simulink model "control_02_flightpath"  (R2020a)
settings: Solver=FixedStepAuto  StartTime=0.0  StopTime=10.0  RelTol=1e-3
model workspace (MAT data in the model file):
  chi = 0.7
  omega = 100
libraries: discretizing x5, simulink x3
settings Model: Creator=Bayram  LastModifiedBy=Julius

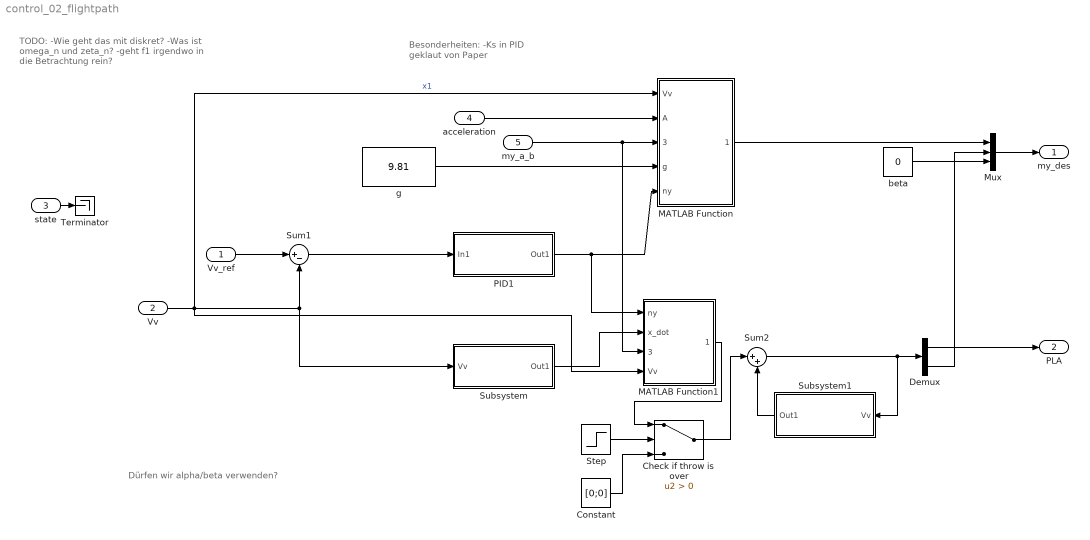
== system control_02_flightpath ==
  note: Dürfen wir alpha/beta verwenden?
  note: Besonderheiten:
      | -Ks in PID geklaut von Paper
  note: TODO:
      | -Wie geht das mit diskret?
      | -Was ist omega_n und zeta_n?
      | -geht f1 irgendwo in die Betrachtung rein?
  Vv_ref : Inport  PortDimensions=3
  Vv : Inport  Port=2  OutDataTypeStr=single  PortDimensions=3
  state : Inport  Port=3  OutDataTypeStr=Bus:fmBus
  acceleration : Inport  Port=4  OutDataTypeStr=single  PortDimensions=3
  my_a_b : Inport  Port=5  OutDataTypeStr=single  PortDimensions=3
  Check if throw is over : Switch  Criteria=u2 > Threshold
  Constant : Constant  Value=[0;0]  OutDataTypeStr=single
  Demux : Demux  Outputs=2
  MATLAB Function : MATLAB Function  TreatAsAtomicUnit=on
  MATLAB Function1 : MATLAB Function  TreatAsAtomicUnit=on
  Mux : Mux  Inputs=3
  PID1 : Subsystem
  Step : Step  Time=7  SampleTime=0
  Subsystem : Subsystem
  Subsystem1 : Subsystem
  Sum1 : Sum  Inputs=|+-
  Sum2 : Sum  Inputs=|++  AccumDataTypeStr=single  OutDataTypeStr=single
  Terminator : Terminator
  beta : Constant  Value=0  OutDataTypeStr=single
  g : Constant  Value=9.81  OutDataTypeStr=double
  my_des : Outport  OutDataTypeStr=single  PortDimensions=3
  PLA : Outport  Port=2  OutDataTypeStr=single  PortDimensions=1
  wires:
  state/1 -> Terminator/1
  MATLAB Function/1(mu_des) -> Mux/1
  Sum2/1 -> Demux/1, Subsystem1/1(Vv)
  Sum1/1 -> PID1/1(In1)
  acceleration/1 -> MATLAB Function/2(A)
  g/1 -> MATLAB Function/4(g)
  PID1/1(Out1) -> MATLAB Function1/1(ny), MATLAB Function/5(ny)
  Vv_ref/1 -> Sum1/1
  Vv/1 -> MATLAB Function/1(Vv), MATLAB Function1/4(Vv), Subsystem/1(Vv), Sum1/2  "x1"
  Subsystem/1(Out1) -> MATLAB Function1/2(x_dot)
  Subsystem1/1(Out1) -> Sum2/2
  my_a_b/1 -> MATLAB Function1/3(my_a_b), MATLAB Function/3(my_a_b)
  beta/1 -> Mux/3
  Mux/1 -> my_des/1
  Demux/1 -> PLA/1
  Demux/2 -> Mux/2
  Constant/1 -> Check if throw is over/3
  Step/1 -> Check if throw is over/2
  MATLAB Function1/1(Delta_x) -> Check if throw is over/1
  Check if throw is over/1 -> Sum2/1

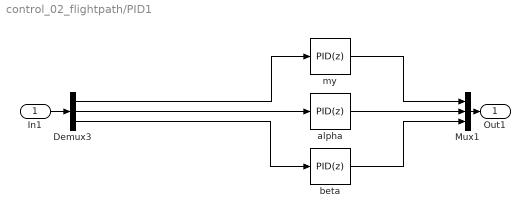
== system control_02_flightpath/PID1 ==
  In1 : Inport
  Demux3 : Demux  Outputs=3
  Mux1 : Mux  Inputs=3
  alpha : simulink/Continuous/PID Controller  Controller=PID  Form=Parallel  TimeDomain=Discrete-time  UseExternalTs=off  SampleTime=-1  IntegratorMethod=Forward Euler  FilterMethod=Forward Euler  ControllerParametersSource=internal  P=1  I=0  D=0  UseFilter=on  N=100  TunerSelectOption=Transfer Function Based (PID Tuner App)  InitialConditionSource=internal  InitialConditionForIntegrator=0  InitialConditionForFilter=0  DifferentiatorICPrevScaledInput=0  ExternalReset=none  TrackingMode=off  Kt=1  LimitOutput=off  UpperSaturationLimit=inf  LowerSaturationLimit=-inf  LinearizeAsGain=off  AntiWindupMode=none  Kb=1  POutMin=[]  POutMax=[]  IOutMin=[]  IOutMax=[]  DOutMin=[]  DOutMax=[]  NOutMin=[]  NOutMax=[]  SumOutMin=[]  SumOutMax=[]  SaturationOutMin=[]  SaturationOutMax=[]  PParamMin=[]  PParamMax=[]  IParamMin=[]  IParamMax=[]  DParamMin=[]  DParamMax=[]  NParamMin=[]  NParamMax=[]  KbParamMin=[]  KbParamMax=[]  KtParamMin=[]  KtParamMax=[]  KbOutMin=[]  KbOutMax=[]  KtOutMin=[]  KtOutMax=[]  IntegratorOutMin=[]  IntegratorOutMax=[]  FilterOutMin=[]  FilterOutMax=[]  SumI1OutMin=[]  SumI1OutMax=[]  SumI2OutMin=[]  SumI2OutMax=[]  SumI3OutMin=[]  SumI3OutMax=[]  SumI4OutMin=[]  SumI4OutMax=[]  SumDOutMin=[]  SumDOutMax=[]  DifferentiatorOutMin=[]  DifferentiatorOutMax=[]  FilterDiffOutCoefMin=[]  FilterDiffOutCoefMax=[]  ReciprocalOutMin=[]  ReciprocalOutMax=[]  SumDenOutMin=[]  SumDenOutMax=[]  SumNumOutMin=[]  SumNumOutMax=[]  DivideOutMin=[]  DivideOutMax=[]  UdiffTsProdOutMin=[]  UdiffTsProdOutMax=[]  NTsProdOutMin=[]  NTsProdOutMax=[]  UintegralTsProdOutMin=[]  UintegralTsProdOutMax=[]  UngainTsProdOutMin=[]  UngainTsProdOutMax=[]  IntegratorContinuousStateAttributes=''  IntegratorStateMustResolveToSignalObject=off  IntegratorRTWStateStorageClass=Auto  FilterContinuousStateAttributes=''  FilterStateMustResolveToSignalObject=off  FilterRTWStateStorageClass=Auto  ParallelPVariant=InternalParameters  IdealPVariant=Disabled  IVariant=InternalParameters  DVariant=InternalParameters  IntegratorVariant=Discrete  SatVariant=Disabled  AWVariant=Passthrough  PCopyVariant=Disabled  TRVariant=Disabled  FdbkBlocksVariant=Forward  IdealPFdbkVariant=Disabled  SatFdbkVariant=Disabled  DerivativeFilterVariant=ForwardEulerFilter  NVariant=InternalParameters  NCopyVariant=Disabled  FilterICVariant=InternalICsFilter  IntegratorICVariant=InternalICs  ExternalResetVariant=Disabled  TRSumVariant=Passthrough  SumFdbkVariant=Disabled  SumVariant=Sum_PID  TsampFilterVariant=InternalTs  TsampNgainVariant=Passthrough  TsampIntegralVariant=Passthrough
  beta : simulink/Continuous/PID Controller  Controller=PID  Form=Parallel  TimeDomain=Discrete-time  UseExternalTs=off  SampleTime=-1  IntegratorMethod=Forward Euler  FilterMethod=Forward Euler  ControllerParametersSource=internal  P=1  I=0  D=0  UseFilter=on  N=100  TunerSelectOption=Transfer Function Based (PID Tuner App)  InitialConditionSource=internal  InitialConditionForIntegrator=0  InitialConditionForFilter=0  DifferentiatorICPrevScaledInput=0  ExternalReset=none  TrackingMode=off  Kt=1  LimitOutput=off  UpperSaturationLimit=inf  LowerSaturationLimit=-inf  LinearizeAsGain=off  AntiWindupMode=none  Kb=1  POutMin=[]  POutMax=[]  IOutMin=[]  IOutMax=[]  DOutMin=[]  DOutMax=[]  NOutMin=[]  NOutMax=[]  SumOutMin=[]  SumOutMax=[]  SaturationOutMin=[]  SaturationOutMax=[]  PParamMin=[]  PParamMax=[]  IParamMin=[]  IParamMax=[]  DParamMin=[]  DParamMax=[]  NParamMin=[]  NParamMax=[]  KbParamMin=[]  KbParamMax=[]  KtParamMin=[]  KtParamMax=[]  KbOutMin=[]  KbOutMax=[]  KtOutMin=[]  KtOutMax=[]  IntegratorOutMin=[]  IntegratorOutMax=[]  FilterOutMin=[]  FilterOutMax=[]  SumI1OutMin=[]  SumI1OutMax=[]  SumI2OutMin=[]  SumI2OutMax=[]  SumI3OutMin=[]  SumI3OutMax=[]  SumI4OutMin=[]  SumI4OutMax=[]  SumDOutMin=[]  SumDOutMax=[]  DifferentiatorOutMin=[]  DifferentiatorOutMax=[]  FilterDiffOutCoefMin=[]  FilterDiffOutCoefMax=[]  ReciprocalOutMin=[]  ReciprocalOutMax=[]  SumDenOutMin=[]  SumDenOutMax=[]  SumNumOutMin=[]  SumNumOutMax=[]  DivideOutMin=[]  DivideOutMax=[]  UdiffTsProdOutMin=[]  UdiffTsProdOutMax=[]  NTsProdOutMin=[]  NTsProdOutMax=[]  UintegralTsProdOutMin=[]  UintegralTsProdOutMax=[]  UngainTsProdOutMin=[]  UngainTsProdOutMax=[]  IntegratorContinuousStateAttributes=''  IntegratorStateMustResolveToSignalObject=off  IntegratorRTWStateStorageClass=Auto  FilterContinuousStateAttributes=''  FilterStateMustResolveToSignalObject=off  FilterRTWStateStorageClass=Auto  ParallelPVariant=InternalParameters  IdealPVariant=Disabled  IVariant=InternalParameters  DVariant=InternalParameters  IntegratorVariant=Discrete  SatVariant=Disabled  AWVariant=Passthrough  PCopyVariant=Disabled  TRVariant=Disabled  FdbkBlocksVariant=Forward  IdealPFdbkVariant=Disabled  SatFdbkVariant=Disabled  DerivativeFilterVariant=ForwardEulerFilter  NVariant=InternalParameters  NCopyVariant=Disabled  FilterICVariant=InternalICsFilter  IntegratorICVariant=InternalICs  ExternalResetVariant=Disabled  TRSumVariant=Passthrough  SumFdbkVariant=Disabled  SumVariant=Sum_PID  TsampFilterVariant=InternalTs  TsampNgainVariant=Passthrough  TsampIntegralVariant=Passthrough
  my : simulink/Continuous/PID Controller  Controller=PID  Form=Parallel  TimeDomain=Discrete-time  UseExternalTs=off  SampleTime=-1  IntegratorMethod=Forward Euler  FilterMethod=Forward Euler  ControllerParametersSource=internal  P=1  I=0  D=0  UseFilter=on  N=100  TunerSelectOption=Transfer Function Based (PID Tuner App)  InitialConditionSource=internal  InitialConditionForIntegrator=0  InitialConditionForFilter=0  DifferentiatorICPrevScaledInput=0  ExternalReset=none  TrackingMode=off  Kt=1  LimitOutput=off  UpperSaturationLimit=inf  LowerSaturationLimit=-inf  LinearizeAsGain=off  AntiWindupMode=none  Kb=1  POutMin=[]  POutMax=[]  IOutMin=[]  IOutMax=[]  DOutMin=[]  DOutMax=[]  NOutMin=[]  NOutMax=[]  SumOutMin=[]  SumOutMax=[]  SaturationOutMin=[]  SaturationOutMax=[]  PParamMin=[]  PParamMax=[]  IParamMin=[]  IParamMax=[]  DParamMin=[]  DParamMax=[]  NParamMin=[]  NParamMax=[]  KbParamMin=[]  KbParamMax=[]  KtParamMin=[]  KtParamMax=[]  KbOutMin=[]  KbOutMax=[]  KtOutMin=[]  KtOutMax=[]  IntegratorOutMin=[]  IntegratorOutMax=[]  FilterOutMin=[]  FilterOutMax=[]  SumI1OutMin=[]  SumI1OutMax=[]  SumI2OutMin=[]  SumI2OutMax=[]  SumI3OutMin=[]  SumI3OutMax=[]  SumI4OutMin=[]  SumI4OutMax=[]  SumDOutMin=[]  SumDOutMax=[]  DifferentiatorOutMin=[]  DifferentiatorOutMax=[]  FilterDiffOutCoefMin=[]  FilterDiffOutCoefMax=[]  ReciprocalOutMin=[]  ReciprocalOutMax=[]  SumDenOutMin=[]  SumDenOutMax=[]  SumNumOutMin=[]  SumNumOutMax=[]  DivideOutMin=[]  DivideOutMax=[]  UdiffTsProdOutMin=[]  UdiffTsProdOutMax=[]  NTsProdOutMin=[]  NTsProdOutMax=[]  UintegralTsProdOutMin=[]  UintegralTsProdOutMax=[]  UngainTsProdOutMin=[]  UngainTsProdOutMax=[]  IntegratorContinuousStateAttributes=''  IntegratorStateMustResolveToSignalObject=off  IntegratorRTWStateStorageClass=Auto  FilterContinuousStateAttributes=''  FilterStateMustResolveToSignalObject=off  FilterRTWStateStorageClass=Auto  ParallelPVariant=InternalParameters  IdealPVariant=Disabled  IVariant=InternalParameters  DVariant=InternalParameters  IntegratorVariant=Discrete  SatVariant=Disabled  AWVariant=Passthrough  PCopyVariant=Disabled  TRVariant=Disabled  FdbkBlocksVariant=Forward  IdealPFdbkVariant=Disabled  SatFdbkVariant=Disabled  DerivativeFilterVariant=ForwardEulerFilter  NVariant=InternalParameters  NCopyVariant=Disabled  FilterICVariant=InternalICsFilter  IntegratorICVariant=InternalICs  ExternalResetVariant=Disabled  TRSumVariant=Passthrough  SumFdbkVariant=Disabled  SumVariant=Sum_PID  TsampFilterVariant=InternalTs  TsampNgainVariant=Passthrough  TsampIntegralVariant=Passthrough
  Out1 : Outport
  wires:
  Mux1/1 -> Out1/1
  In1/1 -> Demux3/1
  my/1 -> Mux1/1
  alpha/1 -> Mux1/2
  beta/1 -> Mux1/3
  Demux3/1 -> my/1
  Demux3/3 -> beta/1
  Demux3/2 -> alpha/1

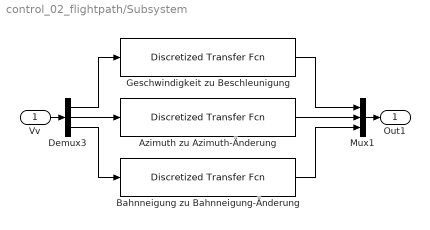
== system control_02_flightpath/Subsystem ==
  Vv : Inport
  Azimuth zu Azimuth-Änderung : discretizing/Discretized Transfer Fcn  Numerator=[(omega)^2]  Denominator=[1 2*(chi)*(omega) (omega)^2]  AbsTol=auto  SampleTime=0.01  method=zoh  Wc=1
      settings: SourceProductBaseCode=SL
  Bahnneigung zu Bahnneigung-Änderung : discretizing/Discretized Transfer Fcn  Numerator=[(omega)^2]  Denominator=[1 2*(chi)*(omega) (omega)^2]  AbsTol=auto  SampleTime=0.01  method=zoh  Wc=1
      settings: SourceProductBaseCode=SL
  Demux3 : Demux  Outputs=3
  Geschwindigkeit zu Beschleunigung : discretizing/Discretized Transfer Fcn  Numerator=[(omega)^2 0]  Denominator=[1 2*(chi)*(omega) (omega)^2]  AbsTol=auto  SampleTime=0.01  method=zoh  Wc=1
      settings: SourceProductBaseCode=SL
  Mux1 : Mux  Inputs=3
  Out1 : Outport
  wires:
  Azimuth zu Azimuth-Änderung/1 -> Mux1/2
  Demux3/3 -> Bahnneigung zu Bahnneigung-Änderung/1
  Bahnneigung zu Bahnneigung-Änderung/1 -> Mux1/3
  Demux3/2 -> Azimuth zu Azimuth-Änderung/1
  Demux3/1 -> Geschwindigkeit zu Beschleunigung/1
  Geschwindigkeit zu Beschleunigung/1 -> Mux1/1
  Vv/1 -> Demux3/1
  Mux1/1 -> Out1/1

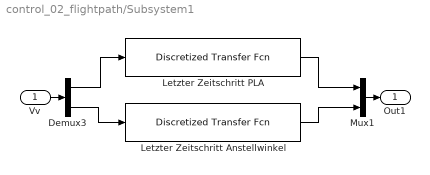
== system control_02_flightpath/Subsystem1 ==
  Vv : Inport  OutDataTypeStr=single  PortDimensions=2
  Demux3 : Demux  Outputs=2
  Letzter Zeitschritt Anstellwinkel : discretizing/Discretized Transfer Fcn  Numerator=[(omega)^2]  Denominator=[1 2*(chi)*(omega) (omega)^2]  AbsTol=auto  SampleTime=0.01  method=zoh  Wc=1
      settings: SourceProductBaseCode=SL
  Letzter Zeitschritt PLA : discretizing/Discretized Transfer Fcn  Numerator=[(omega)^2]  Denominator=[1 2*(chi)*(omega) (omega)^2]  AbsTol=auto  SampleTime=0.01  method=zoh  Wc=1
      settings: SourceProductBaseCode=SL
  Mux1 : Mux  Inputs=2
  Out1 : Outport  OutDataTypeStr=single  PortDimensions=2
  wires:
  Letzter Zeitschritt Anstellwinkel/1 -> Mux1/2
  Demux3/2 -> Letzter Zeitschritt Anstellwinkel/1
  Demux3/1 -> Letzter Zeitschritt PLA/1
  Letzter Zeitschritt PLA/1 -> Mux1/1
  Vv/1 -> Demux3/1
  Mux1/1 -> Out1/1

== matlab function control_02_flightpath/MATLAB Function1 ==
  data: ny input; Delta_x output; x_dot input; my_a_b input; Vv input
function Delta_x = fcn(ny, x_dot, my_a_b, Vv)
    ny = reduce(ny);
    x_dot = reduce(x_dot);
    
    S = 0.468;
    V = Vv(1);
    rho = 1.225;
    q = 0.5*rho*V^2;
    alpha= my_a_b(2);
    my = my_a_b(1);
    m = 4.200;
    
    %initScripts/TromClacl/0degElev (Z = L) (alpha=a)
    C_xPLA = 2.350; %random
    C_xalpha = 0.23011;
    C_zPLA = 0; %random
    C_zalpha = 5.19729;
    
    g = q*S/(m*V)*[V*(C_xPLA *cos(alpha)+C_zPLA*sin(alpha)), V*(C_xalpha*cos(alpha)+C_zalpha*sin(alpha));
                C_xPLA *sin(alpha)*cos(my)-C_zPLA*cos(alpha)*cos(my), C_xalpha*sin(alpha)*cos(my)-C_zalpha*cos(alpha)*cos(my)];
    
    %g_inv = 1 /(g(1,1)*g(2,2) - g(1,2)*g(2,1)) * [ g(2,2), -g(1,2);
    %                                          -g(2,1),  g(1,1)];
Delta_x = g \ (ny-x_dot);

function reduce=reduce(x)
    
    reduce = [0;0];
    reduce(1) = x(1);
    reduce(2) = x(3);
end
    
end

== matlab function control_02_flightpath/MATLAB Function ==
  data: Vv input; A input; my_a_b input; g input; ny input; mu_des output
function mu_des = fcn(Vv, A, my_a_b, g, ny)
    V=Vv(1);
    gamma=Vv(3);
    my=my_a_b(1);
mu_des=atan((ny(2)*V*cos(gamma)-A(2)*cos(my))/(ny(3)*V+A(2)*sin(my)+g*cos(gamma)));
